simulink model "vcu_control"  (R2025a)
settings: Solver=VariableStepAuto  StartTime=0.0  StopTime=10.0  RelTol=1e-3
libraries: drivingvehiclecontroller x2
settings Model: Creator=beatr  LastModifiedBy=beatr

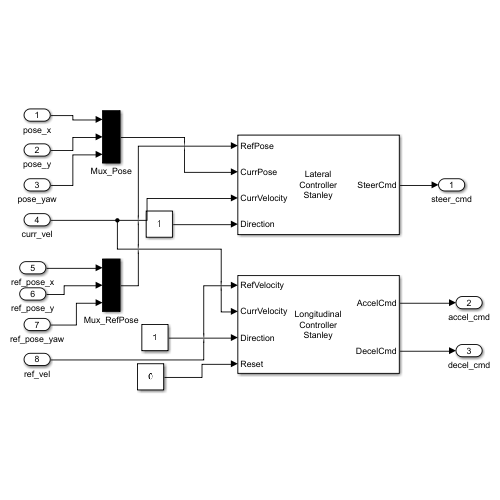
[thumbnail: Simulink's stored preview of the top-level diagram]
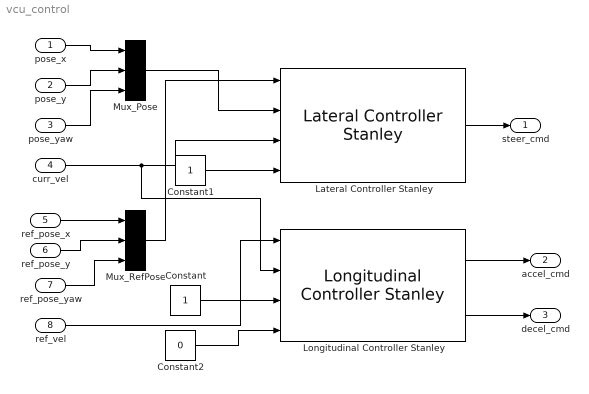
== system vcu_control ==
  pose_x : Inport
  pose_y : Inport  Port=2
  pose_yaw : Inport  Port=3
  curr_vel : Inport  Port=4
  ref_pose_x : Inport  Port=5
  ref_pose_y : Inport  Port=6
  ref_pose_yaw : Inport  Port=7
  ref_vel : Inport  Port=8
  Constant : Constant
  Constant1 : Constant
  Constant2 : Constant  Value=0  OutDataTypeStr=boolean
  Lateral Controller Stanley : drivingvehiclecontroller/Lateral Controller Stanley  ModelType=Kinematic bicycle model  PositionGainF=2.5  PositionGainR=2.5  YawRateGain=0.2  DelayGain=0.2  VehicleMass=1575  Lf=1.2  Lr=1.6  TireStiffness=19000  Wheelbase=2.8  MaxSteeringAngle=35
  Longitudinal Controller Stanley : drivingvehiclecontroller/Longitudinal Controller Stanley  Kp=2.5  Ki=1  SampleTime=0.05  MaxAcceleration=3  MaxDeceleration=6
  Mux_Pose : Mux  Inputs=3
  Mux_RefPose : Mux  Inputs=3
  steer_cmd : Outport
  accel_cmd : Outport  Port=2
  decel_cmd : Outport  Port=3
  wires:
  pose_x/1 -> Mux_Pose/1
  pose_y/1 -> Mux_Pose/2
  pose_yaw/1 -> Mux_Pose/3
  ref_pose_x/1 -> Mux_RefPose/1
  ref_pose_y/1 -> Mux_RefPose/2
  ref_pose_yaw/1 -> Mux_RefPose/3
  curr_vel/1 -> Longitudinal Controller Stanley/2, Lateral Controller Stanley/3
  Lateral Controller Stanley/1 -> steer_cmd/1
  Longitudinal Controller Stanley/1 -> accel_cmd/1
  Longitudinal Controller Stanley/2 -> decel_cmd/1
  Mux_Pose/1 -> Lateral Controller Stanley/2
  Mux_RefPose/1 -> Lateral Controller Stanley/1
  Constant/1 -> Longitudinal Controller Stanley/3
  Constant1/1 -> Lateral Controller Stanley/4
  Constant2/1 -> Longitudinal Controller Stanley/4
  ref_vel/1 -> Longitudinal Controller Stanley/1
